simulink model "JX_Kinect_multi"  (Simulink 7.7)
settings: Solver=ode4  StartTime=0.0  StopTime=inf  FixedStep=sample_time  RelTol=1e-3
InitFcn:
  | sample_time=0.005;%0.004;%0.0025;%0.02;
  | DeltaT = 0.02;
  | g = 9.81;
  | H0 = g%0.3165;
  | Kl = 1;
  | 
  | Omega_r = 1.6;%for Horizontal reference
  | Zeta_r = 1; %for Horizontal reference
  | Omega = 1.8;%for Horizontal Control
  | Zeta = 0.5;    %for Horizontal Control
  | 
  | Omega_h_r = 2.5; %for vertical reference
  | Zeta_h_r = 0.8;  %for vertical reference
  | Omega_h = 2.7;    %for vertical control
  | Zeta_h = 0.8;         %for vertical control
  | PI=pi;
  | 
  | Mass = 1.15;
  | Acc_Max = 4;
  | Acc_Max_h = 4;
  | 
  | Max_RP = 60;
  | 
  | % for NN
  | n = 5;
  | r = 3;
  | n2 = 5;
  | NN_ST = 0.02;
  | 
  | GAMA_V = 6;
  | gama_V_e = 0.01;
  | 
  | GAMA_W = GAMA_V;
  | gama_W_e =0.01;
  | 
  | % deadzone
  | NN_Deadzone_Z = 0;
  | 
  | % inputs nomalizaton parameters
  | NN_Z_y_min = -3;
  | NN_Z_y_max = 0.5;
  | 
  | NN_Z_v_max = 8;
  | NN_Z_v_min = -NN_Z_v_max;
  | 
  | % alpha = 0.034;
  | alpha = 1;
  | % c_f = 0.0015;
  | c_f = 0.001;
  | c_y_tilt = 1*0.5;
  | 
  | %for WK paras
  | Heightcontrol = 0.08;
  | Scale_Factor=1;
  | yoffset=0;
  | 
  | load MaoBi_Oct04_2_int.mat
  | MB_Interp.time = [];
undefined symbols (not defined in the file or in its folder): DiscIntNeverNeededParam
libraries: simulink x14, dspadpt3 x6, X330_Control x4, nid_lib x2
(part 4 of 4)

== matlab function UAV2/Yaw Controller/MATLAB Function ==
  data: u input double; y output double
function y = fcn(u)
%#codegen
y = u;
if y > pi    
    y = y - 2*pi;
elseif y < -pi
        y = y + 2*pi;
end
